simulink model "Copy_of_Model_vertical_lqr"  (R2017b)
settings: Solver=FixedStepAuto  StartTime=0.0  StopTime=10  FixedStep=1e-3  RelTol=1e-3  EnableMultiTasking=on
values from neighbouring files (symbols this model uses):
  a = moment(pwm==0)    [Helicopter_main.m]    (also in Helicopter_main_test.m = moment(pwm==0)/-sin(-0.5223); Lin_simulink.mat = -0.153036; Lin_simulink_test.mat = -0.153036; parametry.m = 0)
  alpha_0 = -28.13    [Helicopter_main.m]    (also in Helicopter_main_test.m = parameters(3); Lin_simulink.mat = -0.522258237308; Lin_simulink_test.mat = -0.52225830565)
  f_v = 0    [Helicopter_main.m]    (also in Helicopter_main_test.m = parameters(2); parametry.m)
  I_v = lsqnonlin(cel, I_v, 0,[],options)    [Helicopter_main.m]    (also in Helicopter_main_test.m; parametry.m = 0)
  J_v = 0    [Helicopter_main.m]    (also in Helicopter_main_test.m = parameters(1); parametry.m)
  K_lqr = lqr(lin_A, lin_B, Q, R, N)    [Helicopter_main_test.m]
  L = place(lin_A.', lin_C.', lambda).'    [Helicopter_main_test.m]
  lin_A = [0 1 0;     a/J_v*cos(lin_alpha_v-alpha_0) -f_v/J_v polyval(lin_M_V_diff, lin_w_v)/J_v;     0 0 -polyval(lin_U_V_diff, lin_w_v)/I_v]    [Helicopter_main_test.m]
  lin_alpha_v = pi/18    (= 0.174532925199)    [Helicopter_main_test.m]
  lin_B = [0; 0; 1/I_v]    [Helicopter_main_test.m]
  lin_C = [1 0 0]    [Helicopter_main_test.m]
  lin_u_v = polyval(wsp_U_V, lin_w_v)    [Helicopter_main_test.m]
  lin_velocity_v = 0    [Helicopter_main_test.m]
  lin_w_v = real(lin_w_v(lin_w_v>-330 & lin_w_v<300 & imag(lin_w_v)==0))    [Helicopter_main_test.m]
  wsp_M_V = polyfit(v/60, moment, 5)    [Helicopter_main.m]    (also in Helicopter_main_test.m = polyfit(v, moment, 5); Lin_simulink.mat = [-2.46242484187e-10 4.61213078344e-09 2.0169387865e-06 1.989; Lin_simulink_test.mat = [-2.51456949125e-14 2.95925329869e-12 8.13117134031e-09 5.04)
  wsp_U_V = polyfit(pred,PWM,5)    [Helicopter_main.m]    (also in Helicopter_main_test.m; Lin_simulink.mat = [-7.28749420126e-10 2.12446681505e-08 6.5068856079e-06 -2.60; Lin_simulink_test.mat = [-7.44181518745e-14 1.363108664e-11 2.62321306545e-08 -6.605)
settings Model: Creator=Student  LastModifiedBy=Marcin
settings DataIOCC: LimitDataPoints=on  SaveFormat=Array
settings OptimizationCC: LifeSpan=inf
settings DebuggingCC: SFUnexpectedBacktrackingDiag=warning  SFNoUnconditionalDefaultTransitionDiag=warning  SFExecutionAtInitializationDiag=none
settings HardwareCC: ProdBitPerPointer=32  ProdBitPerSizeT=32  ProdBitPerPtrDiffT=32  ProdLargestAtomicFloat=None  ProdIntDivRoundTo=Undefined  ProdEndianess=Unspecified  ProdWordSize=32  ProdHWDeviceType=32-bit Generic
settings ModelReferenceCC: PropagateSignalLabelsOutOfModel=off
settings CodeAppCC: StateflowObjectComments=on
settings GRTTargetCC: TargetLangStandard=C89/C90 (ANSI)  GeneratePreprocessorConditionals=Disable all
settings ConfigComp: CovMetricSettings=dw  CovHtmlReporting=on  CovSaveCumulativeToWorkspaceVar=on  CovSaveSingleToWorkspaceVar=on  CovExternalEMLEnable=off

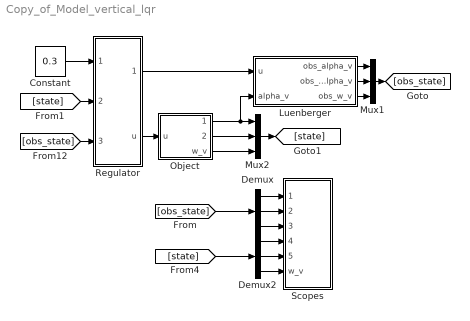
== system Copy_of_Model_vertical_lqr ==
  Constant : Constant  Value=0.3
  Demux : Demux  Outputs=3
  Demux2 : Demux  Outputs=3
  Luenberger : Subsystem
  Mux1 : Mux  Inputs=3
  Mux2 : Mux  Inputs=3
  Object : Subsystem
  Regulator : Subsystem
  Scopes : Subsystem
  wires:
  Object/1(alpha_v) -> Luenberger/2(alpha_v), Mux2/1
  Luenberger/2(obs_dalpha_v) -> Mux1/2
  Luenberger/1(obs_alpha_v) -> Mux1/1
  Luenberger/3(obs_w_v) -> Mux1/3
  Mux1/1 -> [obs_state]
  Mux2/1 -> [state]
  Object/3(w_v) -> Mux2/3
  Object/2(dalpha_v) -> Mux2/2
  Demux/1 -> Scopes/1(obs_alpha_v)
  Demux/2 -> Scopes/2(obs_dalpha_v)
  Demux/3 -> Scopes/3(obs_w_v)
  Demux2/2 -> Scopes/5(dalpha_v)
  Demux2/3 -> Scopes/6(w_v)
  Demux2/1 -> Scopes/4(alpha_v)
  [obs_state] -> Demux/1
  [state] -> Demux2/1
  Constant/1 -> Regulator/1(set point)
  [state] -> Regulator/2(state)
  [obs_state] -> Regulator/3(obs_state)
  Regulator/2(u) -> Object/1(u)
  Regulator/1(obs_u) -> Luenberger/1(u)

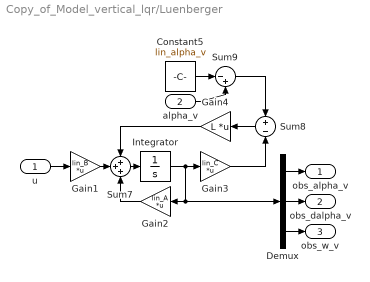
== system Copy_of_Model_vertical_lqr/Luenberger ==
  u : Inport
  alpha_v : Inport  Port=2
  Constant5 : Constant  Value=lin_alpha_v
  Demux : Demux  Outputs=3
  Gain1 : Gain  Gain=lin_B  Multiplication=Matrix(K*u)
  Gain2 : Gain  Gain=lin_A  Multiplication=Matrix(K*u)
  Gain3 : Gain  Gain=lin_C  Multiplication=Matrix(K*u)
  Gain4 : Gain  Gain=L  Multiplication=Matrix(K*u)
  Integrator : Integrator  InitialCondition=[0;0;0]
  Sum7 : Sum  Inputs=+++
  Sum8 : Sum  Inputs=+|-
  Sum9 : Sum  Inputs=|-+
  obs_alpha_v : Outport
  obs_dalpha_v : Outport  Port=2
  obs_w_v : Outport  Port=3
  wires:
  u/1 -> Gain1/1
  alpha_v/1 -> Sum9/2
  Sum7/1 -> Integrator/1
  Gain2/1 -> Sum7/3
  Integrator/1 -> Gain3/1, Demux/1, Gain2/1
  Gain3/1 -> Sum8/2
  Gain1/1 -> Sum7/2
  Sum8/1 -> Gain4/1
  Gain4/1 -> Sum7/1
  Demux/1 -> obs_alpha_v/1
  Demux/2 -> obs_dalpha_v/1
  Demux/3 -> obs_w_v/1
  Constant5/1 -> Sum9/1
  Sum9/1 -> Sum8/1

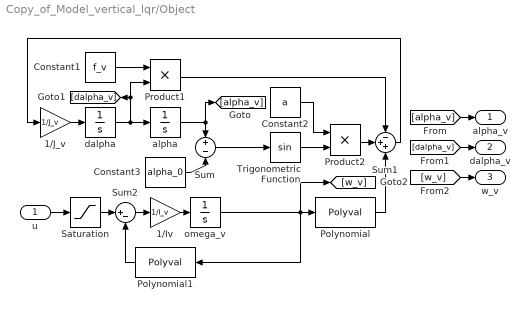
== system Copy_of_Model_vertical_lqr/Object ==
  u : Inport
  1/Iv : Gain  Gain=1/I_v
  1/J_v : Gain  Gain=1/J_v
  Constant1 : Constant  Value=f_v
  Constant2 : Constant  Value=a
  Constant3 : Constant  Value=alpha_0
  Polynomial : Polyval  Coefs=wsp_M_V
  Polynomial1 : Polyval  Coefs=wsp_U_V
  Product1 : Product
  Product2 : Product
  Saturation : Saturate  UpperLimit=1  LowerLimit=-1
  Sum : Sum  Inputs=+|-
  Sum1 : Sum  Inputs=-++
  Sum2 : Sum  Inputs=|+-
  Trigonometric Function : Trigonometry
  alpha : Integrator  InitialCondition=lin_alpha_v+0.1
  dalpha : Integrator  InitialCondition=lin_velocity_v
  omega_v : Integrator  InitialCondition=lin_w_v
  alpha_v : Outport
  dalpha_v : Outport  Port=2
  w_v : Outport  Port=3
  wires:
  dalpha/1 -> [dalpha_v], Product1/2, alpha/1
  Trigonometric Function/1 -> Product2/2
  Polynomial1/1 -> Sum2/2
  Sum/1 -> Trigonometric Function/1
  omega_v/1 -> [w_v], Polynomial1/1, Polynomial/1
  Constant2/1 -> Product2/1
  1/J_v/1 -> dalpha/1
  1/Iv/1 -> omega_v/1
  alpha/1 -> [alpha_v], Sum/1
  Sum2/1 -> 1/Iv/1
  Polynomial/1 -> Sum1/3
  Constant3/1 -> Sum/2
  Product2/1 -> Sum1/2
  Constant1/1 -> Product1/1
  Product1/1 -> Sum1/1
  Sum1/1 -> 1/J_v/1
  Saturation/1 -> Sum2/1
  u/1 -> Saturation/1
  [alpha_v] -> alpha_v/1
  [dalpha_v] -> dalpha_v/1
  [w_v] -> w_v/1

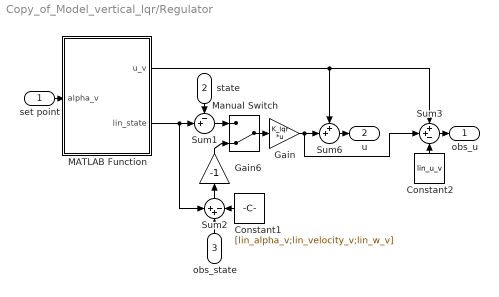
== system Copy_of_Model_vertical_lqr/Regulator ==
  set point : Inport
  state : Inport  Port=2
  obs_state : Inport  Port=3
  Constant1 : Constant  Value=[lin_alpha_v;lin_velocity_v;lin_w_v]
  Constant2 : Constant  Value=lin_u_v
  Gain : Gain  Gain=K_lqr  Multiplication=Matrix(K*u)
  Gain6 : Gain  Gain=-1
  MATLAB Function : MATLAB Function  TreatAsAtomicUnit=on
  Manual Switch : ManualSwitch  CurrentSetting=0
  Sum1 : Sum  Inputs=-+|
  Sum2 : Sum  Inputs=++-
  Sum3 : Sum  Inputs=++-
  Sum6 : Sum  Inputs=++|
  obs_u : Outport
  u : Outport  Port=2
  wires:
  MATLAB Function/1(u_v) -> Sum6/1, Sum3/1
  set point/1 -> MATLAB Function/1(alpha_v)
  Gain6/1 -> Manual Switch/2
  Manual Switch/1 -> Gain/1
  Sum6/1 -> u/1
  Gain/1 -> Sum3/2, Sum6/2
  Sum1/1 -> Manual Switch/1
  obs_state/1 -> Sum2/2
  state/1 -> Sum1/1
  MATLAB Function/2(lin_state) -> Sum2/1, Sum1/2
  Constant1/1 -> Sum2/3
  Sum2/1 -> Gain6/1
  Sum3/1 -> obs_u/1
  Constant2/1 -> Sum3/3

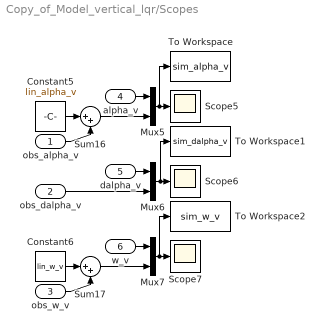
== system Copy_of_Model_vertical_lqr/Scopes ==
  obs_alpha_v : Inport
  obs_dalpha_v : Inport  Port=2
  obs_w_v : Inport  Port=3
  alpha_v : Inport  Port=4
  dalpha_v : Inport  Port=5
  w_v : Inport  Port=6
  Constant5 : Constant  Value=lin_alpha_v
  Constant6 : Constant  Value=lin_w_v
  Mux5 : Mux  Inputs=2
  Mux6 : Mux  Inputs=2
  Mux7 : Mux  Inputs=2
  Scope5 : Scope
  Scope6 : Scope
  Scope7 : Scope
  Sum16 : Sum  Inputs=|++
  Sum17 : Sum  Inputs=|++
  To Workspace : ToWorkspace  VariableName=sim_alpha_v  SampleTime=-1
  To Workspace1 : ToWorkspace  VariableName=sim_dalpha_v  SampleTime=-1
  To Workspace2 : ToWorkspace  VariableName=sim_w_v  SampleTime=-1
  wires:
  Mux7/1 -> To Workspace2/1, Scope7/1
  Sum17/1 -> Mux7/2
  Sum16/1 -> Mux5/2
  Mux5/1 -> To Workspace/1, Scope5/1
  Constant5/1 -> Sum16/1
  alpha_v/1 -> Mux5/1
  dalpha_v/1 -> Mux6/1
  w_v/1 -> Mux7/1
  obs_alpha_v/1 -> Sum16/2
  obs_dalpha_v/1 -> Mux6/2
  Constant6/1 -> Sum17/1
  obs_w_v/1 -> Sum17/2
  Mux6/1 -> To Workspace1/1, Scope6/1

== matlab function Copy_of_Model_vertical_lqr/Regulator/MATLAB Function ==
  data: u_v output double size=1 [0..1]; alpha_v input; lin_state output
function [u_v, lin_state] = Lin(alpha_v)

const = load('Lin_simulink_test.mat');
w_v = roots(const.wsp_M_V+[zeros(1,length(const.wsp_M_V)-1) const.a*sin(alpha_v-const.alpha_0)]);
w_v = real(w_v(w_v>-350 & w_v<350 & imag(w_v)==0));
w_v = w_v(1);
u_v = polyval(const.wsp_U_V, w_v);
u_v = u_v(1);
lin_state = [alpha_v; 0; w_v];
